simulink model "Assign2"  (R2016a)
settings: Solver=FixedStepDiscrete  StartTime=0.0  StopTime=inf  RelTol=1e-3
settings Model: Creator=Muhammed  LastModifiedBy=Muhammed
settings OptimizationCC: DefaultParameterBehavior=Inlined  InlineInvariantSignals=on  EnableMemcpy=off  OptimizeModelRefInitCode=on  LifeSpan=1
settings DebuggingCC: UnderspecifiedInitializationDetection=Classic  MergeDetectMultiDrivingBlocksExec=none
settings ModelReferenceCC: PropagateSignalLabelsOutOfModel=off
settings RTWCC: SystemTargetFile=ert.tlc  GenCodeOnly=on  TemplateMakefile=ert_default_tmf  GenerateReport=on  IncludeHyperlinkInReport=on  LaunchReport=on  GenerateTraceInfo=on  GenerateTraceReport=on  GenerateTraceReportSl=on  GenerateTraceReportSf=on  GenerateTraceReportEml=on
settings CodeAppCC: ForceParamTrailComments=on  IgnoreCustomStorageClasses=off  OperatorAnnotations=on  SimulinkDataObjDesc=on  SFDataObjDesc=on  MATLABFcnDesc=on  InsertBlockDesc=on  MATLABSourceComments=on
settings ERTTargetCC: GenerateSampleERTMain=on  InlinedParameterPlacement=NonHierarchical  ERTCustomFileTemplate=example_file_process.tlc

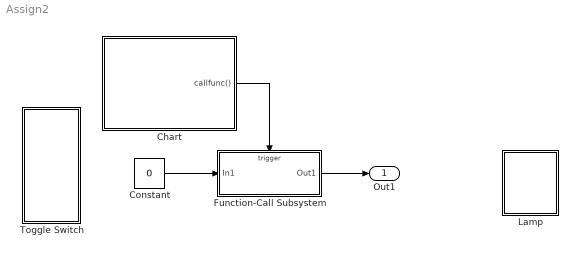
== system Assign2 ==
  Chart : Stateflow chart  TreatAsAtomicUnit=on
  Constant : Constant  Value=0
  Function-Call Subsystem : Subsystem  TreatAsAtomicUnit=on
  Lamp : Subsystem  DialogController=hmiCreateDDGDialog  IsWebBlock=on  mask(MWDashboardBlock){webBlockId=50b24cca-d8f1-4ef6-b9f2-5a07ca5c66c6, webBlockType=lamp, ShowInLibBrowser=on, ShowInitialText=on, HMISrcModelName=Assign2}
      mask prompts: webBlockType "WebBlock Type"; HMISrcModelName "Source Model"
      mask Help: helpview([docroot '/mapfiles/simulink.map'], 'hmi_lamp')
      mask Display:
      | if strcmp(get_param(bdroot(gcb),'BlockDiagramType'), 'library')
      |     image([(matlabroot) '/toolbox/simulink/hmi/icons/Lamp.png']);
      | end
  Toggle Switch : Subsystem  DialogController=hmiCreateDDGDialog  IsWebBlock=on  mask(MWDashboardBlock){webBlockId=6b4e1b19-4e30-4abb-a7c7-b79188c6fe27, webBlockType=toggleswitch, ShowInLibBrowser=on, ShowInitialText=on, HMISrcModelName=Assign2}
      mask prompts: webBlockId "WebBlock Id"; webBlockType "WebBlock Type"; HMISrcModelName "Source Model"
      mask Help: helpview([docroot '/mapfiles/simulink.map'], 'hmi_toggle_switch')
      mask Display:
      | if strcmp(get_param(bdroot(gcb),'BlockDiagramType'), 'library')
      |     image([(matlabroot) '/toolbox/simulink/hmi/icons/ToggleSwitch.png']);
      | end
  Out1 : Outport
  wires:
  Constant/1 -> Function-Call Subsystem/1(In1)
  Function-Call Subsystem/1(Out1) -> Out1/1
  Chart/1(callfunc()) -> Function-Call Subsystem/Trigger

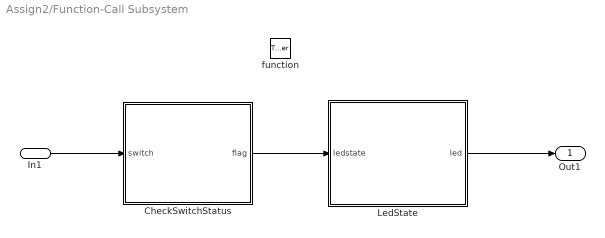
== system Assign2/Function-Call Subsystem ==
  In1 : Inport
  function : TriggerPort  TriggerType=function-call  VariantControl=Variant
  CheckSwitchStatus : Stateflow chart  TreatAsAtomicUnit=on
  "LedState " : Stateflow chart  TreatAsAtomicUnit=on
  Out1 : Outport
  wires:
  In1/1 -> CheckSwitchStatus/1(switch)
  "LedState "/1(led) -> Out1/1
  CheckSwitchStatus/1(flag) -> "LedState "/1(ledstate)

== system Assign2/Lamp ==

== system Assign2/Toggle Switch ==

== stateflow chart Assign2/Function-Call Subsystem/CheckSwitchStatus ==
  (default) -> (junction 7) : % Check Button
  (junction 7) -> (junction 8) [order 1] : [switch == 1 ]
  (junction 7) -> (junction 9) [order 2] : {flag = 0;}
  (junction 8) -> (junction 10) : {flag = 1;}
  (junction 10) -> (junction 9)
  (junction 9) -> (junction 11)
  data: switch input; flag output

== stateflow chart Assign2/Function-Call Subsystem/LedState  ==
  (default) -> (junction 7) : % Led State
  (junction 7) -> (junction 8) [order 1] : [ledstate == 1]
  (junction 7) -> (junction 9) [order 2] : {led = 0 ;}
  (junction 8) -> (junction 10) : {led = 1;}
  (junction 10) -> (junction 9)
  (junction 9) -> (junction 11)
  data: ledstate input double; led output double

== stateflow chart Assign2/Chart ==
  state callFunction
    en:
    du:
    ex:
  (default) -> callFunction
  callFunction -> callFunction : [after(5,msec)]{callfunc;}
  events: callfunc output FUNCTION_CALL_EVENT
